simulink model "exponential_avg_TB"  (R2024a)
settings: Solver=VariableStepAuto  StartTime=0.0  StopTime=1000  RelTol=1e-3
PreLoadFcn:
  | N = 100;
InitFcn:
  | N = 100;
libraries: dspbuff3 x2, dspstat3 x1, dspsrcs4 x1
settings Model: Creator=kschutz  LastModifiedBy=kschutz

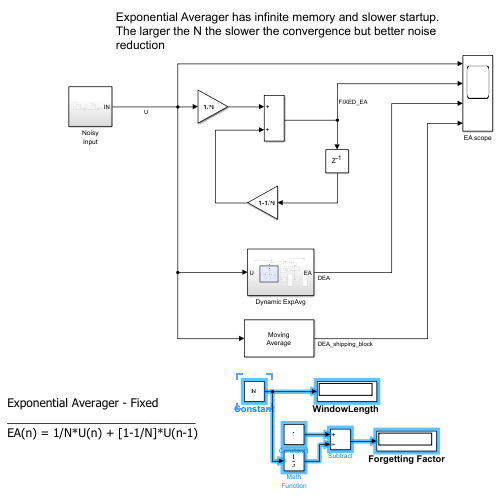
[thumbnail: Simulink's stored preview of the top-level diagram]
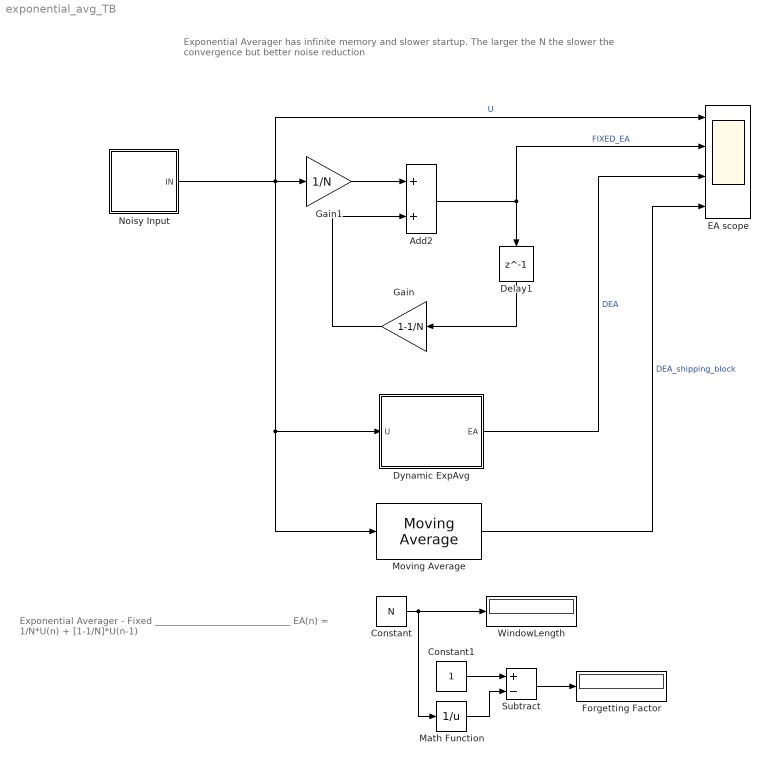
== system exponential_avg_TB ==
  note: Exponential Averager has infinite memory and slower startup.
      | The larger the N the slower the convergence but better noise reduction
  note: Exponential Averager - Fixed
      | _____________________________
      | EA(n) = 1/N*U(n) + [1-1/N]*U(n-1)
  Add2 : Sum
  Constant : Constant  Value=N
  Constant1 : Constant
  Delay1 : Delay  DelayLength=1
  Dynamic ExpAvg : Subsystem
  EA scope : Scope  NumInputPorts=4
  Forgetting Factor : Display
  Gain : Gain  Gain=1-1/N
  Gain1 : Gain  Gain=1/N
  Math Function : Math  Operator=reciprocal
  Moving Average : dspstat3/Moving Average  Method=Exponential weighting  ForgettingFactorPort=off  SpecifyWindowLength=on  WindowLength=N  OverlapLength=15  AllowArbitraryInputLength=off  ForgettingFactor=1-1/N  SimulateUsing=Interpreted execution
  Noisy Input : Subsystem
  Subtract : Sum  Inputs=+-
  "WindowLength " : Display
  wires:
  Gain1/1 -> Add2/1
  Gain/1 -> Add2/2
  Delay1/1 -> Gain/1
  Noisy Input/1(IN) -> EA scope/1, Dynamic ExpAvg/1(U), Moving Average/1, Gain1/1  "U"
  Add2/1 -> EA scope/2, Delay1/1  "FIXED_EA"
  Dynamic ExpAvg/1(EA) -> EA scope/3  "DEA"
  Moving Average/1 -> EA scope/4  "DEA_shipping_block"
  Constant/1 -> "WindowLength "/1, Math Function/1
  Math Function/1 -> Subtract/2
  Constant1/1 -> Subtract/1
  Subtract/1 -> Forgetting Factor/1

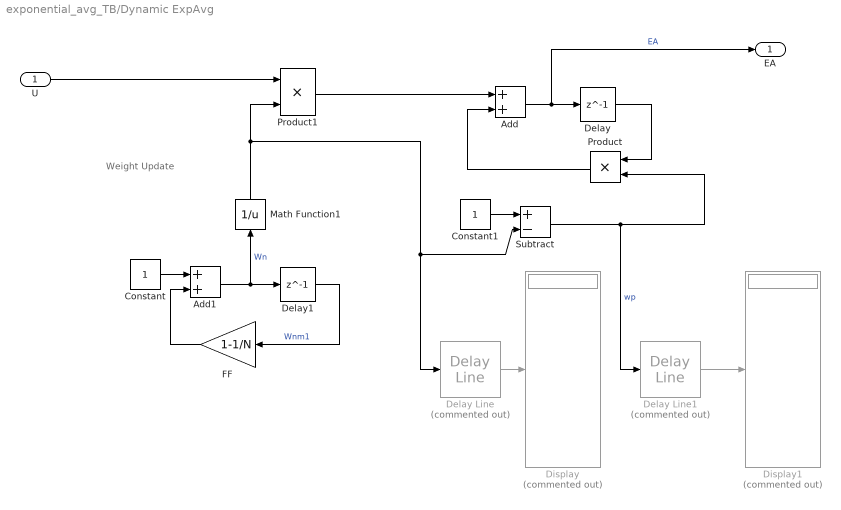
== system exponential_avg_TB/Dynamic ExpAvg ==
  note: Weight Update
  U : Inport
  Add : Sum
  Add1 : Sum
  Constant : Constant  SampleTime=1
  Constant1 : Constant
  Delay : Delay  DelayLength=1
  Delay Line : dspbuff3/Delay Line  Commented=on  siz=10  ic=0  directfeed=on  enable_output=off  hold_output=off  OutputFrames=off
  Delay Line1 : dspbuff3/Delay Line  Commented=on  siz=10  ic=0  directfeed=on  enable_output=off  hold_output=off  OutputFrames=off
  Delay1 : Delay  DelayLength=1
  Display : Display  Commented=on
  Display1 : Display  Commented=on
  FF : Gain  Gain=1-1/N
  Math Function1 : Math  Operator=reciprocal
  Product : Product
  Product1 : Product
  Subtract : Sum  Inputs=+-
  EA : Outport
  wires:
  Constant/1 -> Add1/1
  Delay1/1 -> FF/1  "Wnm1"
  Add1/1 -> Delay1/1, Math Function1/1  "Wn"
  Add/1 -> EA/1, Delay/1  "EA"
  Product1/1 -> Add/1
  Delay/1 -> Product/1
  Math Function1/1 -> Product1/2, Delay Line/1, Subtract/2
  Constant1/1 -> Subtract/1
  Subtract/1 -> Product/2, Delay Line1/1  "wp"
  FF/1 -> Add1/2
  Product/1 -> Add/2
  U/1 -> Product1/1
  Delay Line/1 -> Display/1
  Delay Line1/1 -> Display1/1

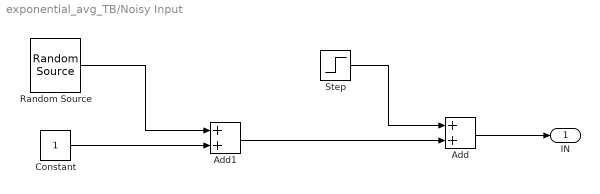
== system exponential_avg_TB/Noisy Input ==
  Add : Sum
  Add1 : Sum
  Constant : Constant  SampleTime=1
  Random Source : dspsrcs4/Random Source  SrcType=Gaussian  MinVal=0  MaxVal=1  MeanVal=0  VarVal=.2  RepMode=Specify seed  rawSeed=123  IsInherit=off  SampTime=1  SampFrame=1  OutComplex=Real  DataType=double  SimulateUsing=Interpreted execution
  Step : Step  Time=500  SampleTime=0
  IN : Outport  VectorParamsAs1DForOutWhenUnconnected=off
  wires:
  Constant/1 -> Add1/2
  Random Source/1 -> Add1/1
  Add/1 -> IN/1
  Add1/1 -> Add/2
  Step/1 -> Add/1
